simulink model "power_netsim1"  (Simulink 6.0)
settings: Solver=ode15s  SolverMode=SingleTasking  StartTime=0.0  StopTime=0.1  RelTol=1e-3  AbsTol=0.01
libraries: powerlib x10
settings Model: Creator=patrice  LastModifiedBy=batserve  ExtModeTrigMode=oneshot  ExtModeArmWhenConnect=off  ExtModeAutoUpdateStatusClock=off
settings SolverCC: MaxOrder=2
settings DataIOCC: LimitDataPoints=off  SignalLoggingName=sigsOut
settings OptimizationCC: BooleanDataType=off
settings DebuggingCC: SolverPrmCheckMsg=none
settings HardwareCC: TargetUnknown=on
settings RTWCC: TemplateMakefile=grt_unix.tmf

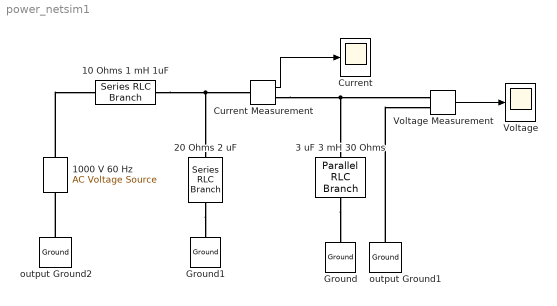
== system power_netsim1 ==
  10 Ohms 1 mH 1uF : powerlib/Elements/Series RLC Branch  PhysicalDomain=powersysdomain  SubClassName=unknown  PortType=p1  LConnTagsString=__new0  RConnTagsString=__new0  Resistance=10  Inductance=1e-03  Capacitance=1e-06  Measurements=None
  1000 V 60 Hz : powerlib/Electrical Sources/AC Voltage Source  Description=source block  Orientation=up  Amplitude=1000  Phase=0  Frequency=60  SampleTime=0  Measurements=None
      settings: AttributesFormatString=\n
  20 Ohms 2 uF : powerlib/Elements/Series RLC Branch  Orientation=down  PhysicalDomain=powersysdomain  SubClassName=unknown  PortType=p1  LConnTagsString=__new0  RConnTagsString=__new0  Resistance=20  Inductance=0  Capacitance=2e-06  Measurements=None
  3 uF 3 mH 30 Ohms : powerlib/Elements/Parallel RLC Branch  Orientation=down  PhysicalDomain=powersysdomain  SubClassName=unknown  PortType=p1  LConnTagsString=a  RConnTagsString=__new0  Resistance=30  Inductance=3e-03  Capacitance=3e-06  Measurements=None
  Current : Scope
      settings: TickLabels=on  YMin=-0.5  YMax=0.5  DataFormat=Array  MaxDataPoints=100000
  Current Measurement : powerlib/Measurements/Current Measurement  Tag=PoWeRsYsTeMmEaSuReMeNt  PhasorSimulation=off  OutputType=Magnitude  PSBequivalent=0
  Ground : powerlib/Elements/Ground  Orientation=down  PhysicalDomain=powersysdomain  SubClassName=unknown  PortType=p1  LConnTagsString=a  RConnTagsString=__newr0
  Ground1 : powerlib/Elements/Ground  Orientation=down  PhysicalDomain=powersysdomain  SubClassName=unknown  PortType=p1  LConnTagsString=a  RConnTagsString=__newr0
  Voltage : Scope
      settings: TickLabels=on  YMin=-0.5  YMax=0.5  DataFormat=Array  MaxDataPoints=100000
  Voltage Measurement : powerlib/Measurements/Voltage Measurement  Tag=PoWeRsYsTeMmEaSuReMeNt  PhasorSimulation=off  OutputType=Magnitude  PSBequivalent=0
  output Ground1 : powerlib/Elements/Ground  Orientation=down  PhysicalDomain=powersysdomain  SubClassName=unknown  PortType=p1  LConnTagsString=a  RConnTagsString=__newr0
  output Ground2 : powerlib/Elements/Ground  Orientation=down  PhysicalDomain=powersysdomain  SubClassName=unknown  PortType=p1  LConnTagsString=a  RConnTagsString=__newr0
  wires:
  Current Measurement/1 -> Current/1
  Voltage Measurement/1 -> Voltage/1
  connections:
  output Ground2/LConn1 -- 1000 V 60 Hz/LConn1
  1000 V 60 Hz/RConn1 -- 10 Ohms 1 mH 1uF/LConn1
  20 Ohms 2 uF/RConn1 -- Ground1/LConn1
  3 uF 3 mH 30 Ohms/RConn1 -- Ground/LConn1
  10 Ohms 1 mH 1uF/RConn1 -- 20 Ohms 2 uF/LConn1 -- Current Measurement/LConn1
  Current Measurement/RConn1 -- 3 uF 3 mH 30 Ohms/LConn1 -- Voltage Measurement/LConn1
  output Ground1/LConn1 -- Voltage Measurement/LConn2
